simulink model "basic_disc"  (Simulink 5.0)
settings: Solver=ode45  StartTime=t_init  StopTime=t_final  RelTol=1e-3
values from neighbouring files (symbols this model uses):
  A = axes('FontSize',fs)    [axesprop.m]    (also in seshft.m = [A zeros(Arows,Bcols-Acols)])
  B = -B    [left_prm.m]    (also in myc2d.m = num(first_nz:length(num)); seshft.m = [B zeros(Brows,Acols-Bcols)])
undefined symbols (not defined in the file or in its folder): gamma, Rc, Sc, st, Tc, Ts, zk
settings Model: Creator=kannan  LastModifiedBy=kannan  ExtModeAutoUpdateStatusClock=off

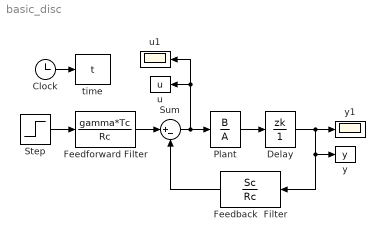
== system basic_disc ==
  Clock : Clock
      settings: Decimation=10
  Delay : DiscreteFilter  Numerator=zk  Denominator=1  SampleTime=Ts
  Feedback  Filter : DiscreteFilter  Orientation=left  Numerator=Sc  Denominator=Rc  SampleTime=Ts
  Feedforward Filter : DiscreteFilter  Numerator=gamma*Tc  Denominator=Rc  SampleTime=Ts
  Plant : DiscreteFilter  Numerator=B  Denominator=A  SampleTime=Ts
  Step : Step  Time=0  After=st  SampleTime=Ts
  Sum : Sum  Inputs=|+-  SaturateOnIntegerOverflow=on
  time : ToWorkspace  VariableName=t  SampleTime=Ts  SaveFormat=Array
  u : ToWorkspace  VariableName=u  SampleTime=Ts  SaveFormat=Array
  u1 : Scope
      settings: YMin=-6e+164  YMax=1.02293e+149
  y : ToWorkspace  VariableName=y  SampleTime=Ts  SaveFormat=Array
  y1 : Scope
      settings: YMin=-6e+164  YMax=1.02293e+149
  wires:
  Feedforward Filter/1 -> Sum/1
  Feedback  Filter/1 -> Sum/2
  Clock/1 -> time/1
  Sum/1 -> u1/1, u/1, Plant/1
  Plant/1 -> Delay/1
  Step/1 -> Feedforward Filter/1
  Delay/1 -> y1/1, Feedback  Filter/1, y/1
